simulink model "car_model"  (R2025b)
settings: Solver=ode4  StartTime=0.0  StopTime=T_sim  FixedStep=0.001  RelTol=1e-3
undefined symbols (not defined in the file): c, k, m, Ts
libraries: simulink_extras x1
settings Model: Creator=Abhay  LastModifiedBy=Abhay

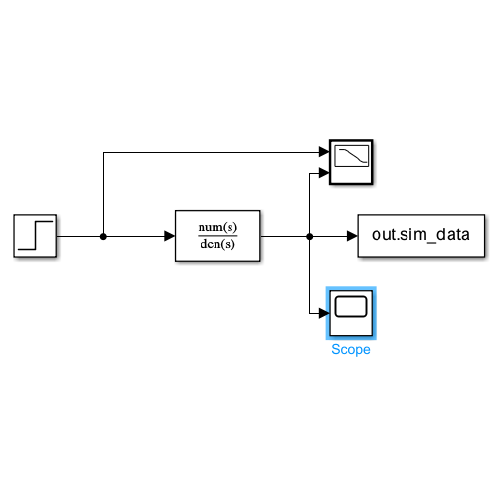
[thumbnail: Simulink's stored preview of the top-level diagram]
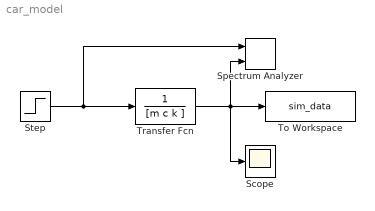
== system car_model ==
  Scope : Scope
      settings: ActiveDisplayYMinimum=-5.5056936519179453E-7  ActiveDisplayYMaximum=1.0200024775004585E-5
  Spectrum Analyzer : simulink_extras/Additional Sinks/Spectrum Analyzer  npts=256  fftpts=256  HowOften=64  sampleT=0.1
  Step : Step  After=0.1  SampleTime=0
  To Workspace : ToWorkspace  VariableName=sim_data  SampleTime=Ts
  Transfer Fcn : TransferFcn  Denominator=[m c k ]
  wires:
  Step/1 -> Spectrum Analyzer/1, Transfer Fcn/1
  Transfer Fcn/1 -> Scope/1, Spectrum Analyzer/2, To Workspace/1
